simulink model "SImulation_Motor"  (R2023a)
settings: Solver=VariableStepAuto  StartTime=0.0  StopTime=10.0  RelTol=1e-3
undefined symbols (not defined in the file): B, J, Kb, kt, La, Ra
libraries: fuzblock x3
settings Model: Creator=dania  LastModifiedBy=Arham khan
settings SolverCC: AlgebraicLoopSolver=TrustRegion
settings DebuggingCC: UnconnectedInputMsg=warning  UnconnectedOutputMsg=warning  UnconnectedLineMsg=warning
settings ModelReferenceCC: EnableRefExpFcnMdlSchedulingChecks=on

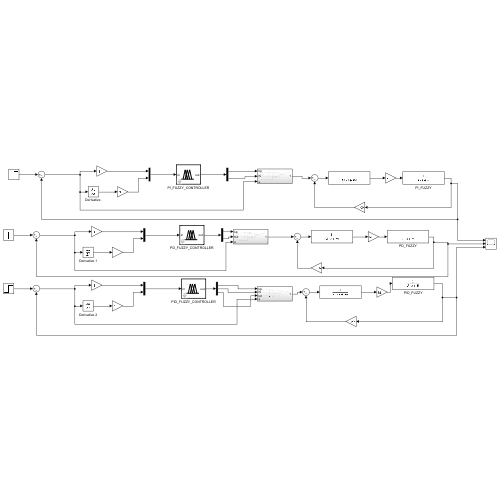
[thumbnail: Simulink's stored preview of the top-level diagram]
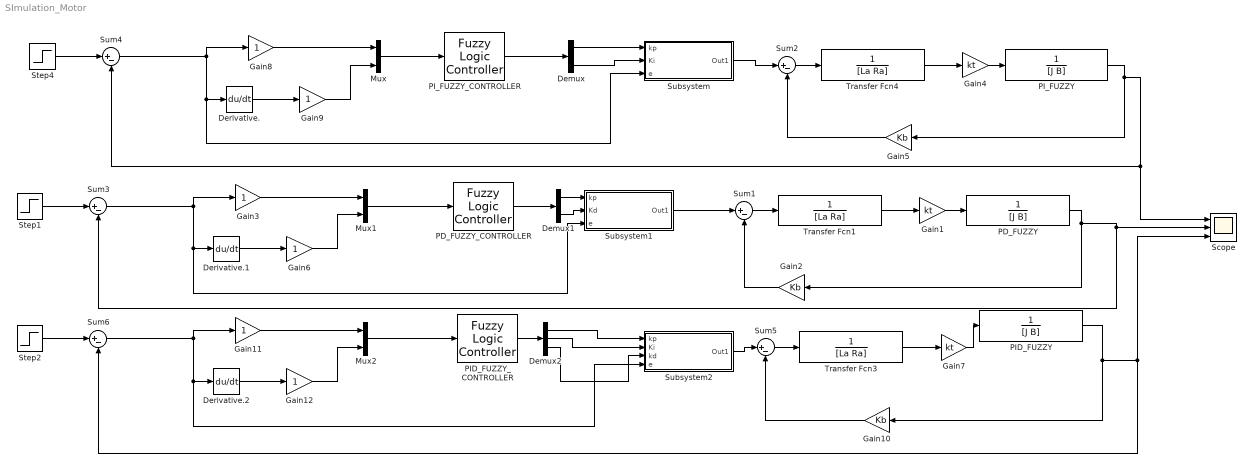
== system SImulation_Motor ==
  Demux : Demux  Outputs=2
  Demux1 : Demux  Outputs=2
  Demux2 : Demux  Outputs=3
  Derivative. : Derivative
  Derivative.1 : Derivative
  Derivative.2 : Derivative
  Gain1 : Gain  Gain=kt
  Gain10 : Gain  Gain=Kb
  Gain{3,6,8..9,11..12} (6 alike) : Gain
  Gain2 : Gain  Gain=Kb
  Gain4 : Gain  Gain=kt
  Gain5 : Gain  Gain=Kb
  Gain7 : Gain  Gain=kt
  Mux : Mux  Inputs=2
  Mux1 : Mux  Inputs=2
  Mux2 : Mux  Inputs=2
  PD_FUZZY : TransferFcn  Denominator=[J B]
  PD_FUZZY_CONTROLLER : fuzblock/Fuzzy Logic  Controller  FIS='PD_control.fis'  OutputSampleNumber=101  DataType=double  FuzzifiedInputs=off  RuleFiringStrengths=off  RuleOutputs=off  AggregatedOutputs=off  SimulateUsing=Interpreted execution  OutOfRangeInputValueMessage=warning  NoRuleFiredMessage=warning  EmptyOutputFuzzySetMessage=warning
  PID_FUZZY : TransferFcn  Denominator=[J B]
  PID_FUZZY_CONTROLLER : fuzblock/Fuzzy Logic  Controller  FIS='PID_control.fis'  OutputSampleNumber=101  DataType=double  FuzzifiedInputs=off  RuleFiringStrengths=off  RuleOutputs=off  AggregatedOutputs=off  SimulateUsing=Interpreted execution  OutOfRangeInputValueMessage=warning  NoRuleFiredMessage=warning  EmptyOutputFuzzySetMessage=warning
  PI_FUZZY : TransferFcn  Denominator=[J B]
  PI_FUZZY_CONTROLLER : fuzblock/Fuzzy Logic  Controller  FIS='PI_control.fis'  OutputSampleNumber=101  DataType=double  FuzzifiedInputs=off  RuleFiringStrengths=off  RuleOutputs=off  AggregatedOutputs=off  SimulateUsing=Interpreted execution  OutOfRangeInputValueMessage=warning  NoRuleFiredMessage=warning  EmptyOutputFuzzySetMessage=warning
  Scope : Scope  NumInputPorts=3
  Step1 : Step  SampleTime=0
  Step2 : Step  SampleTime=0
  Step4 : Step  SampleTime=0
  Subsystem : Subsystem
  Subsystem1 : Subsystem
  Subsystem2 : Subsystem
  Sum{1..6} (6 alike) : Sum  Inputs=|+-
  Transfer Fcn1 : TransferFcn  Denominator=[La Ra]
  Transfer Fcn3 : TransferFcn  Denominator=[La Ra]
  Transfer Fcn4 : TransferFcn  Denominator=[La Ra]
  wires:
  Gain8/1 -> Mux/1
  Sum4/1 -> Gain8/1, Subsystem/3(e), Derivative./1
  Mux/1 -> PI_FUZZY_CONTROLLER/1
  Derivative./1 -> Gain9/1
  Step4/1 -> Sum4/1
  Gain9/1 -> Mux/2
  PI_FUZZY_CONTROLLER/1 -> Demux/1
  Gain5/1 -> Sum2/2
  Gain4/1 -> PI_FUZZY/1
  Subsystem/1(Out1) -> Sum2/1
  Sum2/1 -> Transfer Fcn4/1
  Transfer Fcn4/1 -> Gain4/1
  PI_FUZZY/1 -> Gain5/1, Scope/1, Sum4/2
  Demux/1 -> Subsystem/1(kp)
  Demux1/1 -> Subsystem1/1(kp)
  Gain2/1 -> Sum1/2
  Gain1/1 -> PD_FUZZY/1
  PD_FUZZY/1 -> Gain2/1, Scope/2, Sum3/2
  Transfer Fcn1/1 -> Gain1/1
  Sum1/1 -> Transfer Fcn1/1
  Subsystem1/1(Out1) -> Sum1/1
  PD_FUZZY_CONTROLLER/1 -> Demux1/1
  Step1/1 -> Sum3/1
  Gain6/1 -> Mux1/2
  Sum3/1 -> Gain3/1, Subsystem1/3(e), Derivative.1/1
  Mux1/1 -> PD_FUZZY_CONTROLLER/1
  Derivative.1/1 -> Gain6/1
  Gain3/1 -> Mux1/1
  Demux2/1 -> Subsystem2/1(kp)
  Gain10/1 -> Sum5/2
  Gain7/1 -> PID_FUZZY/1
  PID_FUZZY/1 -> Gain10/1, Scope/3, Sum6/2
  Transfer Fcn3/1 -> Gain7/1
  Sum5/1 -> Transfer Fcn3/1
  Subsystem2/1(Out1) -> Sum5/1
  PID_FUZZY_CONTROLLER/1 -> Demux2/1
  Step2/1 -> Sum6/1
  Gain12/1 -> Mux2/2
  Sum6/1 -> Gain11/1, Subsystem2/4(e), Derivative.2/1
  Mux2/1 -> PID_FUZZY_CONTROLLER/1
  Derivative.2/1 -> Gain12/1
  Gain11/1 -> Mux2/1
  Demux/2 -> Subsystem/2(Ki)
  Demux1/2 -> Subsystem1/2(Kd)
  Demux2/3 -> Subsystem2/3(kd)
  Demux2/2 -> Subsystem2/2(Ki)

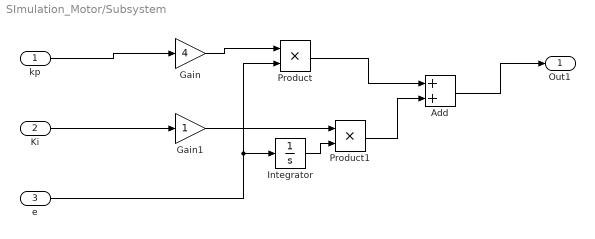
== system SImulation_Motor/Subsystem ==
  kp : Inport
  Ki : Inport  Port=2
  e : Inport  Port=3
  Add : Sum
  Gain : Gain  Gain=4
  Gain1 : Gain
  Integrator : Integrator
  Product : Product
  Product1 : Product
  Out1 : Outport
  wires:
  e/1 -> Integrator/1, Product/2
  Ki/1 -> Gain1/1
  Gain1/1 -> Product1/1
  Integrator/1 -> Product1/2
  Gain/1 -> Product/1
  kp/1 -> Gain/1
  Product/1 -> Add/1
  Product1/1 -> Add/2
  Add/1 -> Out1/1

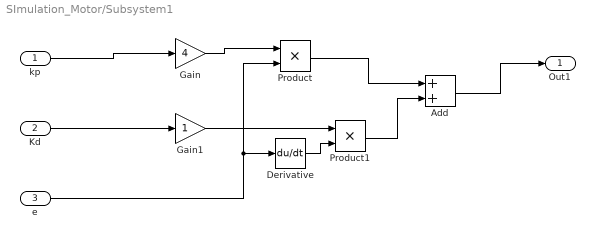
== system SImulation_Motor/Subsystem1 ==
  kp : Inport
  Kd : Inport  Port=2
  e : Inport  Port=3
  Add : Sum
  Derivative : Derivative
  Gain : Gain  Gain=4
  Gain1 : Gain
  Product : Product
  Product1 : Product
  Out1 : Outport
  wires:
  Kd/1 -> Gain1/1
  Gain1/1 -> Product1/1
  e/1 -> Derivative/1, Product/2
  Gain/1 -> Product/1
  kp/1 -> Gain/1
  Product/1 -> Add/1
  Product1/1 -> Add/2
  Add/1 -> Out1/1
  Derivative/1 -> Product1/2

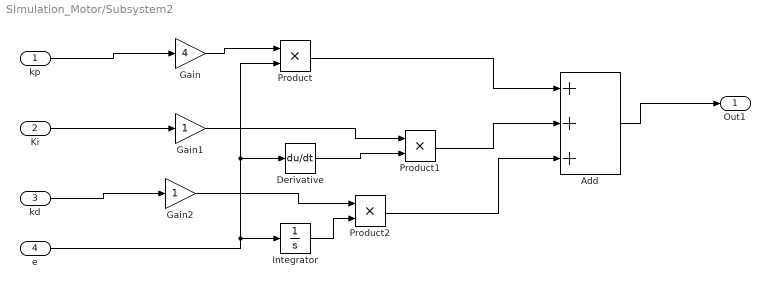
== system SImulation_Motor/Subsystem2 ==
  kp : Inport
  Ki : Inport  Port=2
  kd : Inport  Port=3
  e : Inport  Port=4
  Add : Sum  Inputs=+++
  Derivative : Derivative
  Gain : Gain  Gain=4
  Gain1 : Gain
  Gain2 : Gain
  Integrator : Integrator
  Product : Product
  Product1 : Product
  Product2 : Product
  Out1 : Outport
  wires:
  Gain/1 -> Product/1
  kp/1 -> Gain/1
  Product/1 -> Add/1
  Product1/1 -> Add/2
  Add/1 -> Out1/1
  e/1 -> Integrator/1, Derivative/1, Product/2
  Ki/1 -> Gain1/1
  Gain1/1 -> Product1/1
  kd/1 -> Gain2/1
  Gain2/1 -> Product2/1
  Integrator/1 -> Product2/2
  Derivative/1 -> Product1/2
  Product2/1 -> Add/3
